simulink model "CSE1_HIL_full16_caseC_new_param"  (R2018b)
settings: Solver=VariableStepAuto  StartTime=0.0  StopTime=300  MaxStep=10e-3  RelTol=1e-3
settings Model: Creator=einarsu  LastModifiedBy=martin
settings OptimizationCC: LifeSpan=inf
settings DebuggingCC: SFExecutionAtInitializationDiag=none
settings SFSimCC: SimUseLocalCustomCode=off
settings RTWCC: RTWUseLocalCustomCode=off
settings CodeAppCC: StateflowObjectComments=on

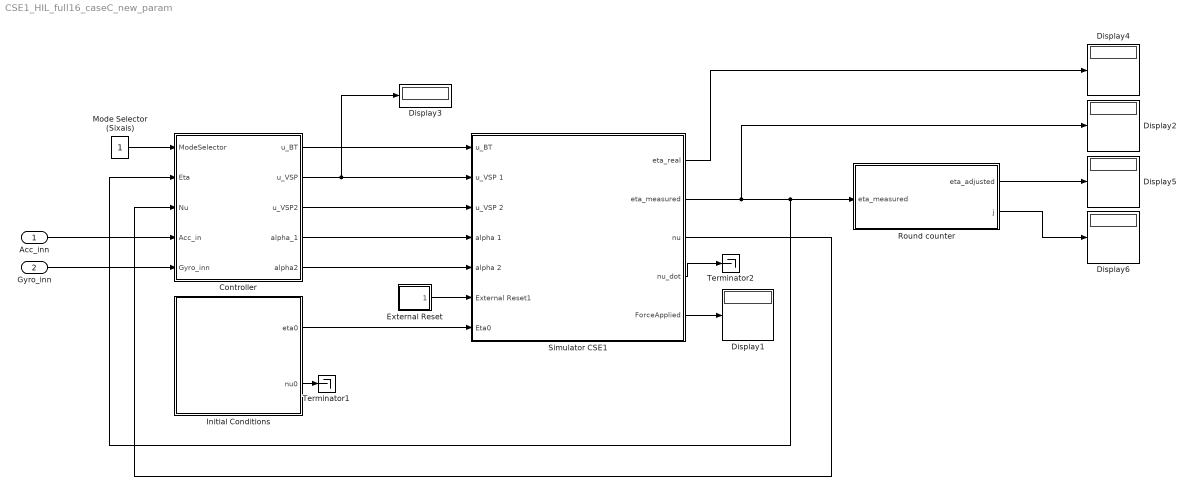
== system CSE1_HIL_full16_caseC_new_param ==
  Acc_inn : Inport
  Gyro_inn : Inport  Port=2
  Controller : Subsystem
  Display{1..6} (6 alike) : Display
  External Reset : Subsystem
  "Initial Conditions " : Subsystem
  Mode Selector (Sixais) : Constant
  Round counter : Subsystem
  Simulator CSE1 : Subsystem
  Terminator1 : Terminator
  Terminator2 : Terminator
  wires:
  Controller/1(u_BT) -> Simulator CSE1/1(u_BT)
  Controller/4(alpha_1) -> Simulator CSE1/4(alpha 1)
  Controller/2(u_VSP) -> Display3/1, Simulator CSE1/2(u_VSP 1)
  Controller/5(alpha2) -> Simulator CSE1/5(alpha 2)
  Controller/3("u_VSP2 ") -> Simulator CSE1/3(u_VSP 2)
  External Reset/1(Out1) -> Simulator CSE1/6(External Reset1)
  "Initial Conditions "/1(eta0) -> Simulator CSE1/7(Eta0)
  Mode Selector (Sixais)/1 -> Controller/1(ModeSelector)
  Simulator CSE1/2(eta_measured) -> Display2/1, Controller/2(Eta), Round counter/1(eta_measured)
  Acc_inn/1 -> Controller/4(Acc_in)
  Gyro_inn/1 -> Controller/5(Gyro_inn)
  Simulator CSE1/5(ForceApplied) -> Display1/1
  "Initial Conditions "/2(nu0) -> Terminator1/1
  Simulator CSE1/4(nu_dot) -> Terminator2/1
  Simulator CSE1/3(nu) -> Controller/3(Nu)
  Simulator CSE1/1(eta_real) -> Display4/1
  Round counter/1(eta_adjusted) -> Display5/1
  Round counter/2(j) -> Display6/1

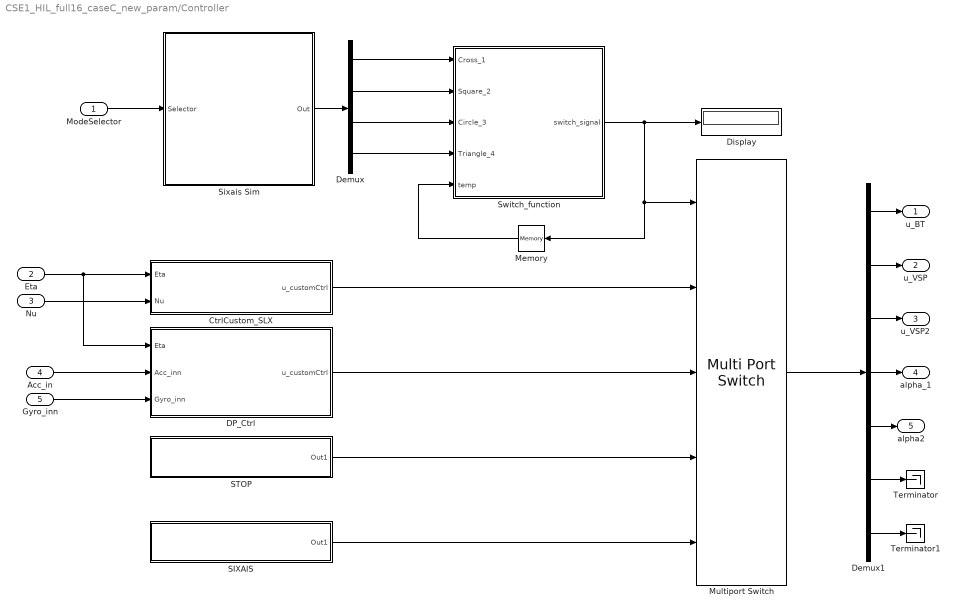
== system CSE1_HIL_full16_caseC_new_param/Controller ==
  ModeSelector : Inport
  Eta : Inport  Port=2
  Nu : Inport  Port=3
  Acc_in : Inport  Port=4
  Gyro_inn : Inport  Port=5
  CtrlCustom_SLX : Subsystem
  DP_Ctrl : Subsystem
  Demux : Demux
  Demux1 : Demux  Outputs=7
  Display : Display
  Memory : Memory  InitialCondition=4
  Multiport Switch : MultiPortSwitch  Inputs=4
  SIXAIS : Subsystem
  STOP : Subsystem
  Sixais Sim : MATLAB Function  TreatAsAtomicUnit=on
  Switch_function : MATLAB Function  TreatAsAtomicUnit=on
  Terminator : Terminator
  Terminator1 : Terminator
  u_BT : Outport
  u_VSP : Outport  Port=2
  "u_VSP2 " : Outport  Port=3
  alpha_1 : Outport  Port=4
  alpha2 : Outport  Port=5
  wires:
  Memory/1 -> Switch_function/5(temp)
  CtrlCustom_SLX/1(u_customCtrl) -> Multiport Switch/2
  Demux/1 -> Switch_function/1(Cross_1)
  Demux/2 -> Switch_function/2(Square_2)
  Demux/3 -> Switch_function/3(Circle_3)
  Demux/4 -> Switch_function/4(Triangle_4)
  Sixais Sim/1(Out) -> Demux/1
  ModeSelector/1 -> Sixais Sim/1(Selector)
  STOP/1(Out1) -> Multiport Switch/4
  SIXAIS/1(Out1) -> Multiport Switch/5
  Eta/1 -> DP_Ctrl/1(Eta), CtrlCustom_SLX/1(Eta)
  Multiport Switch/1 -> Demux1/1
  Demux1/1 -> u_BT/1
  Demux1/2 -> u_VSP/1
  Demux1/3 -> "u_VSP2 "/1
  Demux1/4 -> alpha_1/1
  Demux1/5 -> alpha2/1
  Demux1/6 -> Terminator/1
  Demux1/7 -> Terminator1/1
  Acc_in/1 -> DP_Ctrl/2(Acc_inn)
  Gyro_inn/1 -> DP_Ctrl/3(Gyro_inn)
  DP_Ctrl/1(u_customCtrl) -> Multiport Switch/3
  Switch_function/1(switch_signal) -> Display/1, Memory/1, Multiport Switch/1
  Nu/1 -> CtrlCustom_SLX/2(Nu)

== system CSE1_HIL_full16_caseC_new_param/External Reset ==
  note: Most relevant for Real-Time Simulations...
  Constant : Constant  Value=0
  Out1 : Outport
  wires:
  Constant/1 -> Out1/1

== system CSE1_HIL_full16_caseC_new_param/Initial Conditions  ==
  Eta0 : Constant  Value=[0, 0, 0]'
  "V0 " : Constant  Value=zeros(3,1)
  eta0 : Outport
  nu0 : Outport  Port=2
  wires:
  "V0 "/1 -> nu0/1
  Eta0/1 -> eta0/1

== system CSE1_HIL_full16_caseC_new_param/Round counter ==
  eta_measured : Inport
  Memory : Memory  InitialCondition=[0 0 0]'
  Memory1 : Memory
  Round counter : MATLAB Function  TreatAsAtomicUnit=on
  eta_adjusted : Outport
  j : Outport  Port=2
  wires:
  eta_measured/1 -> Round counter/1(eta_measured)
  Round counter/1(eta_adjusted) -> eta_adjusted/1
  Memory/1 -> Round counter/2(eta_measured_prev)
  Round counter/2(eta_measured_new) -> Memory/1
  Memory1/1 -> Round counter/3(j_prev)
  Round counter/3(j_new) -> Memory1/1, j/1

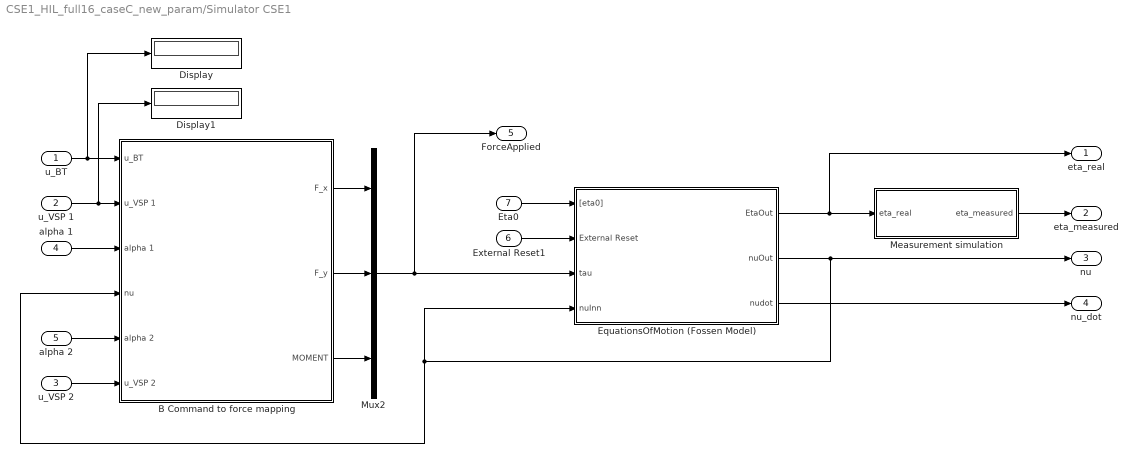
== system CSE1_HIL_full16_caseC_new_param/Simulator CSE1 ==
  u_BT : Inport
  u_VSP 1 : Inport  Port=2
  u_VSP 2 : Inport  Port=3
  alpha 1 : Inport  Port=4
  alpha 2 : Inport  Port=5
  External Reset1 : Inport  Port=6
  Eta0 : Inport  Port=7
  B Command to force mapping : Subsystem
  Display : Display
  Display1 : Display
  EquationsOfMotion (Fossen Model) : Subsystem
  Measurement simulation : MATLAB Function  TreatAsAtomicUnit=on
  Mux2 : Mux  Inputs=3
  eta_real : Outport
  eta_measured : Outport  Port=2
  nu : Outport  Port=3
  nu_dot : Outport  Port=4
  ForceApplied : Outport  Port=5
  wires:
  alpha 2/1 -> B Command to force mapping/5(alpha 2)
  B Command to force mapping/2("F_y ") -> Mux2/2
  B Command to force mapping/1(F_x) -> Mux2/1
  u_VSP 1/1 -> Display1/1, B Command to force mapping/2(u_VSP 1)
  alpha 1/1 -> B Command to force mapping/3(alpha 1)
  u_BT/1 -> Display/1, B Command to force mapping/1(u_BT)
  u_VSP 2/1 -> B Command to force mapping/6(u_VSP 2)
  EquationsOfMotion (Fossen Model)/2(nuOut) -> B Command to force mapping/4(nu), EquationsOfMotion (Fossen Model)/4(nuInn), nu/1
  Eta0/1 -> EquationsOfMotion (Fossen Model)/1("[eta0] ")
  External Reset1/1 -> EquationsOfMotion (Fossen Model)/2(External Reset)
  EquationsOfMotion (Fossen Model)/3(nudot) -> nu_dot/1
  B Command to force mapping/3("MOMENT ") -> Mux2/3
  Mux2/1 -> ForceApplied/1, EquationsOfMotion (Fossen Model)/3(tau)
  EquationsOfMotion (Fossen Model)/1(EtaOut) -> eta_real/1, Measurement simulation/1(eta_real)
  Measurement simulation/1(eta_measured) -> eta_measured/1

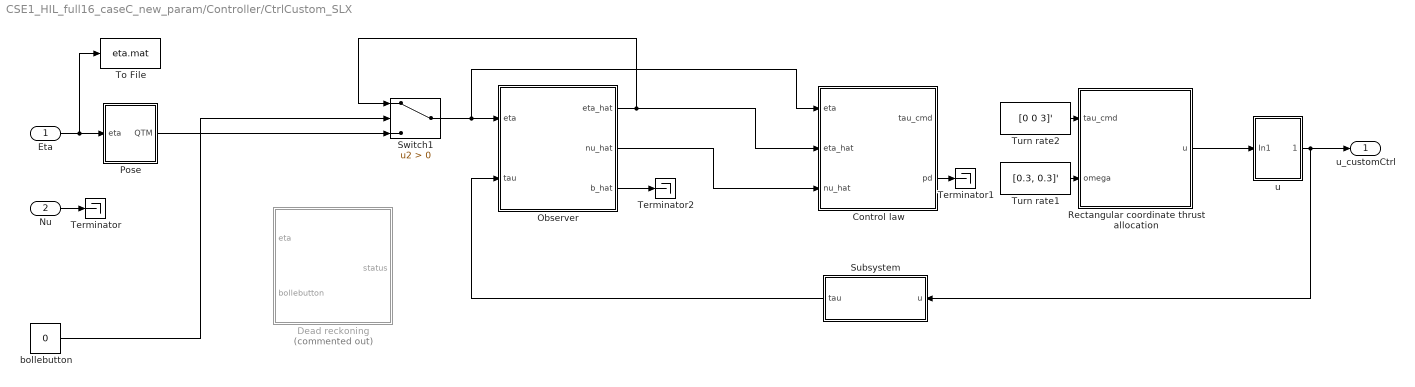
== system CSE1_HIL_full16_caseC_new_param/Controller/CtrlCustom_SLX ==
  Eta : Inport
  Nu : Inport  Port=2
  Control law : Subsystem
  Dead reckoning : Subsystem  Commented=on
  Observer : Subsystem
  Pose : Subsystem
  Rectangular coordinate thrust allocation : Subsystem
  Subsystem : Subsystem
  Switch1 : Switch  Criteria=u2 > Threshold
  Terminator : Terminator
  Terminator1 : Terminator
  Terminator2 : Terminator
  To File : ToFile  Filename=eta.mat  MatrixName=eta
  Turn rate1 : Constant  Value=[0.3, 0.3]'  VectorParams1D=off
  Turn rate2 : Constant  Value=[0 0 3]'  VectorParams1D=off
  bollebutton : Constant  Value=0
  u : Subsystem
  u_customCtrl : Outport
  wires:
  Turn rate1/1 -> Rectangular coordinate thrust allocation/2("omega ")
  Eta/1 -> To File/1, Pose/1(eta)
  u/1(Out1) -> Subsystem/1(u), u_customCtrl/1
  Rectangular coordinate thrust allocation/1(u) -> u/1(In1)
  bollebutton/1 -> Switch1/2
  Pose/1(QTM) -> Switch1/3
  Switch1/1 -> Observer/1(eta), Control law/1(eta)
  Observer/1(eta_hat) -> Control law/2(eta_hat), Switch1/1
  Subsystem/1(tau) -> Observer/2(tau)
  Nu/1 -> Terminator/1
  Observer/2("nu_hat ") -> Control law/3(nu_hat)
  Control law/2(pd) -> Terminator1/1
  Observer/3(b_hat) -> Terminator2/1
  Turn rate2/1 -> Rectangular coordinate thrust allocation/1(tau_cmd)

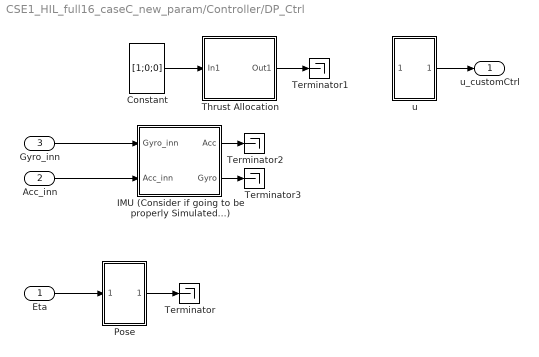
== system CSE1_HIL_full16_caseC_new_param/Controller/DP_Ctrl ==
  Eta : Inport
  Acc_inn : Inport  Port=2
  Gyro_inn : Inport  Port=3
  Constant : Constant  Value=[1;0;0]
  IMU (Consider if going to be properly Simulated...) : Subsystem
  Pose : Subsystem
  Terminator{,1..3} (4 alike) : Terminator
  "Thrust Allocation " : Subsystem
  u : Subsystem
  u_customCtrl : Outport
  wires:
  Pose/1(QTM) -> Terminator/1
  Gyro_inn/1 -> IMU (Consider if going to be properly Simulated...)/1(Gyro_inn)
  Acc_inn/1 -> IMU (Consider if going to be properly Simulated...)/2(Acc_inn)
  Eta/1 -> Pose/1(eta)
  u/1(Out1) -> u_customCtrl/1
  Constant/1 -> "Thrust Allocation "/1(In1)
  "Thrust Allocation "/1(Out1) -> Terminator1/1
  IMU (Consider if going to be properly Simulated...)/1(Acc) -> Terminator2/1
  IMU (Consider if going to be properly Simulated...)/2(Gyro) -> Terminator3/1

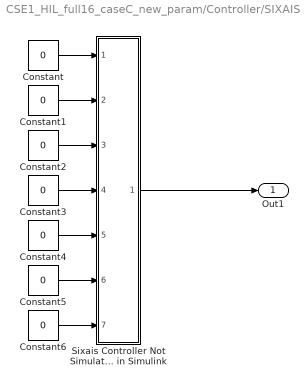
== system CSE1_HIL_full16_caseC_new_param/Controller/SIXAIS ==
  Constant{,1..6} (7 alike) : Constant  Value=0
  Sixais Controller Not Simulated in Simulink : Subsystem
  Out1 : Outport
  wires:
  Constant/1 -> Sixais Controller Not Simulated in Simulink/1(In1)
  Constant1/1 -> Sixais Controller Not Simulated in Simulink/2(In2)
  Constant2/1 -> Sixais Controller Not Simulated in Simulink/3(In3)
  Constant3/1 -> Sixais Controller Not Simulated in Simulink/4(In4)
  Constant4/1 -> Sixais Controller Not Simulated in Simulink/5(In5)
  Constant5/1 -> Sixais Controller Not Simulated in Simulink/6(In6)
  Constant6/1 -> Sixais Controller Not Simulated in Simulink/7(In7)
  Sixais Controller Not Simulated in Simulink/1(Out1) -> Out1/1

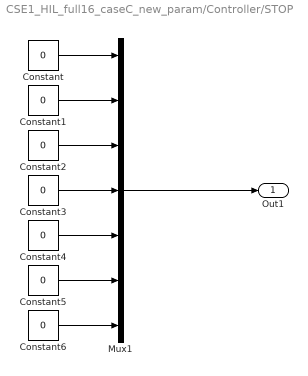
== system CSE1_HIL_full16_caseC_new_param/Controller/STOP ==
  Constant{,1..6} (7 alike) : Constant  Value=0
  Mux1 : Mux  Inputs=7
  Out1 : Outport
  wires:
  Mux1/1 -> Out1/1
  Constant/1 -> Mux1/1
  Constant1/1 -> Mux1/2
  Constant2/1 -> Mux1/3
  Constant3/1 -> Mux1/4
  Constant4/1 -> Mux1/5
  Constant5/1 -> Mux1/6
  Constant6/1 -> Mux1/7

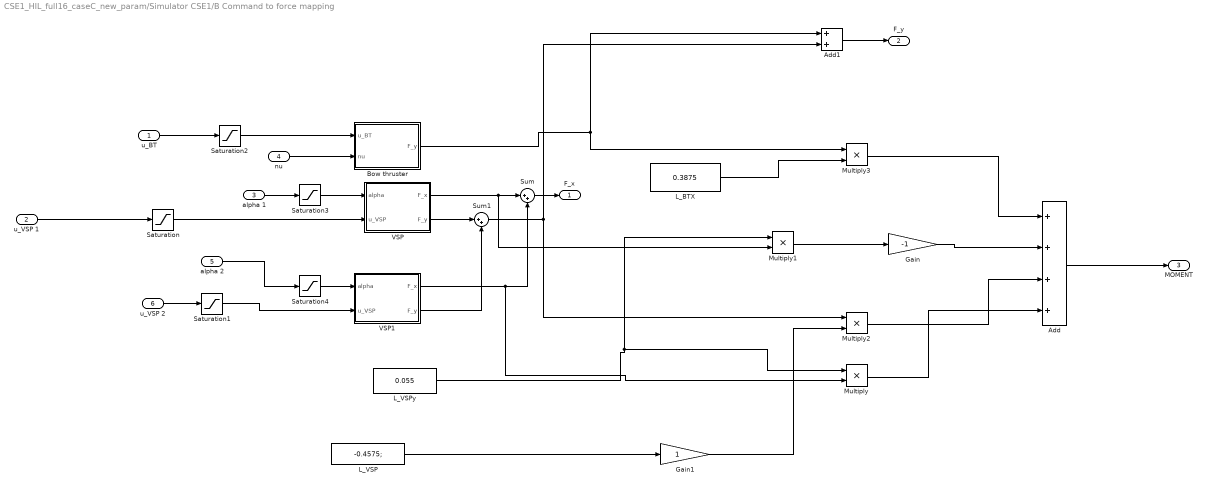
== system CSE1_HIL_full16_caseC_new_param/Simulator CSE1/B Command to force mapping ==
  u_BT : Inport
  u_VSP 1 : Inport  Port=2
  alpha 1 : Inport  Port=3
  nu : Inport  Port=4
  alpha 2 : Inport  Port=5
  u_VSP 2 : Inport  Port=6
  Add : Sum  Inputs=++++
  Add1 : Sum
  Bow thruster : MATLAB Function  TreatAsAtomicUnit=on
  Gain : Gain  Gain=-1
  Gain1 : Gain
  L_BTX : Constant  Value=0.3875
  L_VSP : Constant  Value=-0.4575;
  L_VSPy : Constant  Value=0.055
  Multiply{,1..3} (4 alike) : Product
  Saturation : Saturate  UpperLimit=1  LowerLimit=0
  Saturation1 : Saturate  UpperLimit=1  LowerLimit=0
  Saturation2 : Saturate  UpperLimit=1  LowerLimit=-1
  Saturation3 : Saturate  UpperLimit=pi  LowerLimit=-pi
  Saturation4 : Saturate  UpperLimit=pi  LowerLimit=-pi
  Sum : Sum  Inputs=|++
  Sum1 : Sum  Inputs=|++
  VSP : MATLAB Function  TreatAsAtomicUnit=on
  VSP1 : MATLAB Function  TreatAsAtomicUnit=on
  F_x : Outport
  "F_y " : Outport  Port=2
  "MOMENT " : Outport  Port=3
  wires:
  alpha 1/1 -> Saturation3/1
  nu/1 -> Bow thruster/2(nu)
  Bow thruster/1(F_y) -> Add1/1, Multiply3/1
  VSP/2(F_y) -> Sum1/1
  Sum1/1 -> Add1/2, Multiply2/1
  VSP1/2(F_y) -> Sum1/2
  VSP1/1(F_x) -> Multiply/2, Sum/2
  VSP/1(F_x) -> Multiply1/2, Sum/1
  Sum/1 -> F_x/1
  alpha 2/1 -> Saturation4/1
  u_VSP 2/1 -> Saturation1/1
  L_VSP/1 -> Gain1/1
  L_BTX/1 -> Multiply3/2
  L_VSPy/1 -> Multiply/1, Multiply1/1
  Multiply3/1 -> Add/1
  Multiply1/1 -> Gain/1
  Multiply2/1 -> Add/3
  Multiply/1 -> Add/4
  Add/1 -> "MOMENT "/1
  Gain/1 -> Add/2
  Gain1/1 -> Multiply2/2
  Add1/1 -> "F_y "/1
  Saturation/1 -> VSP/2(u_VSP)
  Saturation1/1 -> VSP1/2(u_VSP)
  u_BT/1 -> Saturation2/1
  u_VSP 1/1 -> Saturation/1
  Saturation2/1 -> Bow thruster/1(u_BT)
  Saturation3/1 -> VSP/1(alpha)
  Saturation4/1 -> VSP1/1(alpha)

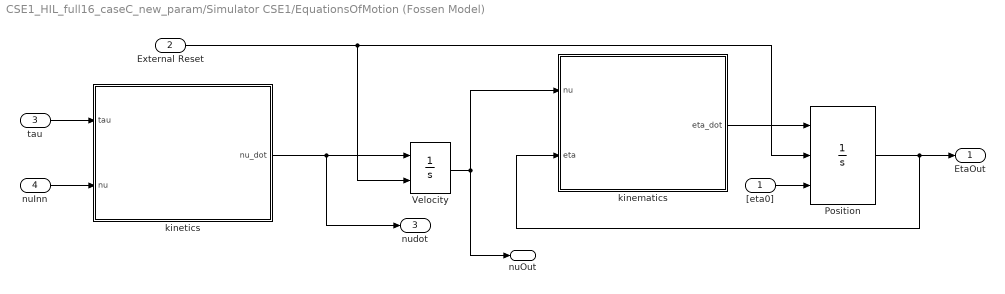
== system CSE1_HIL_full16_caseC_new_param/Simulator CSE1/EquationsOfMotion (Fossen Model) ==
  "[eta0] " : Inport
  External Reset : Inport  Port=2
  tau : Inport  Port=3
  nuInn : Inport  Port=4
  Position : Integrator  ExternalReset=either  InitialConditionSource=external  InitialCondition=[0 0 0]'
  Velocity : Integrator  ExternalReset=either  InitialCondition=[0 0 0]'
  kinematics : MATLAB Function  TreatAsAtomicUnit=on
  kinetics : MATLAB Function  TreatAsAtomicUnit=on
  EtaOut : Outport
  nuOut : Outport  Port=2
  nudot : Outport  Port=3
  wires:
  tau/1 -> kinetics/1(tau)
  Position/1 -> kinematics/2(eta), EtaOut/1
  "[eta0] "/1 -> Position/3
  nuInn/1 -> kinetics/2(nu)
  kinematics/1(eta_dot) -> Position/1
  Velocity/1 -> kinematics/1(nu), nuOut/1
  kinetics/1(nu_dot) -> nudot/1, Velocity/1
  External Reset/1 -> Position/2, Velocity/2

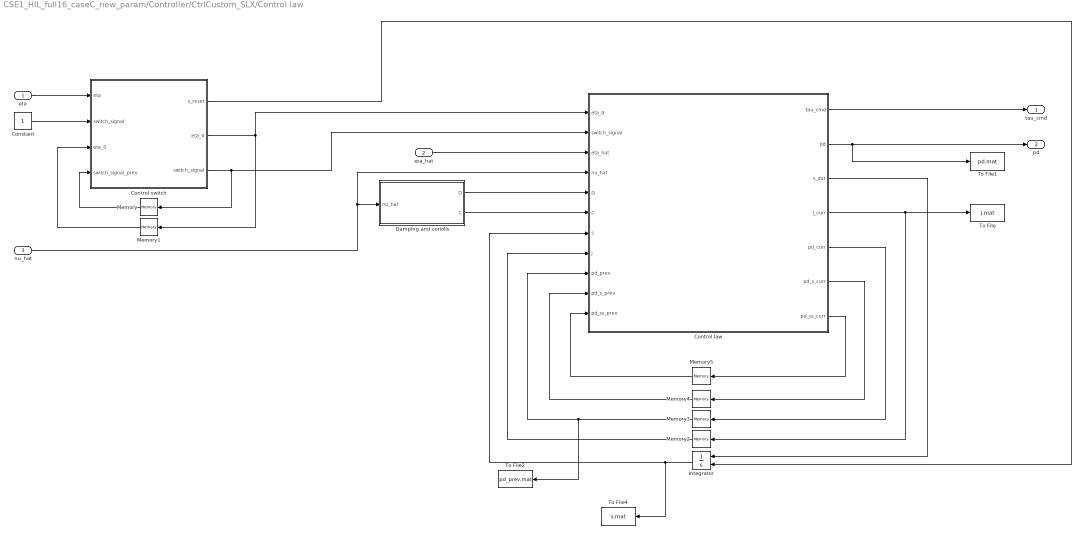
== system CSE1_HIL_full16_caseC_new_param/Controller/CtrlCustom_SLX/Control law ==
  eta : Inport
  eta_hat : Inport  Port=2
  nu_hat : Inport  Port=3
  " Control switch" : MATLAB Function  TreatAsAtomicUnit=on
  Constant : Constant
  Control law : MATLAB Function  TreatAsAtomicUnit=on
  Damping and coriolis : MATLAB Function  TreatAsAtomicUnit=on
  Integrator : Integrator  ExternalReset=either
  Memory : Memory
  Memory1 : Memory  InitialCondition=[0, 0, 0]'
  Memory2 : Memory
  Memory3 : Memory  InitialCondition=[0;0;0]
  Memory4 : Memory  InitialCondition=[0;0;0]
  Memory5 : Memory  InitialCondition=[0;0;0]
  To File : ToFile  Filename=j.mat  MatrixName=j
  To File1 : ToFile  Filename=pd.mat  MatrixName=pd
  To File2 : ToFile  Filename=pd_prev.mat  MatrixName=pd_prev
  To File4 : ToFile  Filename=s.mat  MatrixName=s
  tau_cmd : Outport
  pd : Outport  Port=2
  wires:
  " Control switch"/2(eta_0) -> Memory1/1, Control law/1(eta_0)
  Integrator/1 -> To File4/1, Control law/7(s)
  Damping and coriolis/1(D) -> Control law/5(D)
  Control law/3(s_dot) -> Integrator/1
  Memory1/1 -> " Control switch"/3("eta_0 ")
  " Control switch"/3(switch_signal) -> Memory/1, Control law/2(switch_signal)
  Memory/1 -> " Control switch"/4(switch_signal_prev)
  eta/1 -> " Control switch"/1(eta)
  Constant/1 -> " Control switch"/2("switch_signal ")
  Control law/2(pd) -> To File1/1, pd/1
  Control law/1(tau_cmd) -> tau_cmd/1
  nu_hat/1 -> Damping and coriolis/1(nu_hat), Control law/4(nu_hat)
  Control law/4(j_curr) -> Memory2/1, To File/1
  Memory2/1 -> Control law/8(j)
  Memory3/1 -> Control law/9(pd_prev), To File2/1
  Control law/5(pd_curr) -> Memory3/1
  Damping and coriolis/2(C) -> Control law/6(C)
  eta_hat/1 -> Control law/3(eta_hat)
  Control law/6(pd_s_curr) -> Memory4/1
  Control law/7(pd_ss_curr) -> Memory5/1
  Memory5/1 -> Control law/11(pd_ss_prev)
  Memory4/1 -> Control law/10(pd_s_prev)
  " Control switch"/1(s_reset) -> Integrator/2

== system CSE1_HIL_full16_caseC_new_param/Controller/CtrlCustom_SLX/Dead reckoning ==
  eta : Inport
  bollebutton : Inport  Port=2
  Display : Display
  Memory : Memory  InitialCondition=[0 0 0]'
  Memory1 : Memory  InitialCondition=[0 0 0]'
  Memory2 : Memory  InitialCondition=[0 0 0]'
  dead_reckoning : MATLAB Function  TreatAsAtomicUnit=on
  status : Outport
  wires:
  Memory2/1 -> dead_reckoning/3("last ")
  Memory/1 -> dead_reckoning/5("last3 ")
  dead_reckoning/3(last2) -> Memory1/1
  dead_reckoning/4(last3) -> Memory/1
  Memory1/1 -> dead_reckoning/4("last2 ")
  dead_reckoning/2(last) -> Memory2/1
  eta/1 -> dead_reckoning/1(eta)
  bollebutton/1 -> dead_reckoning/2(bollebutton)
  dead_reckoning/1(status) -> Display/1, status/1

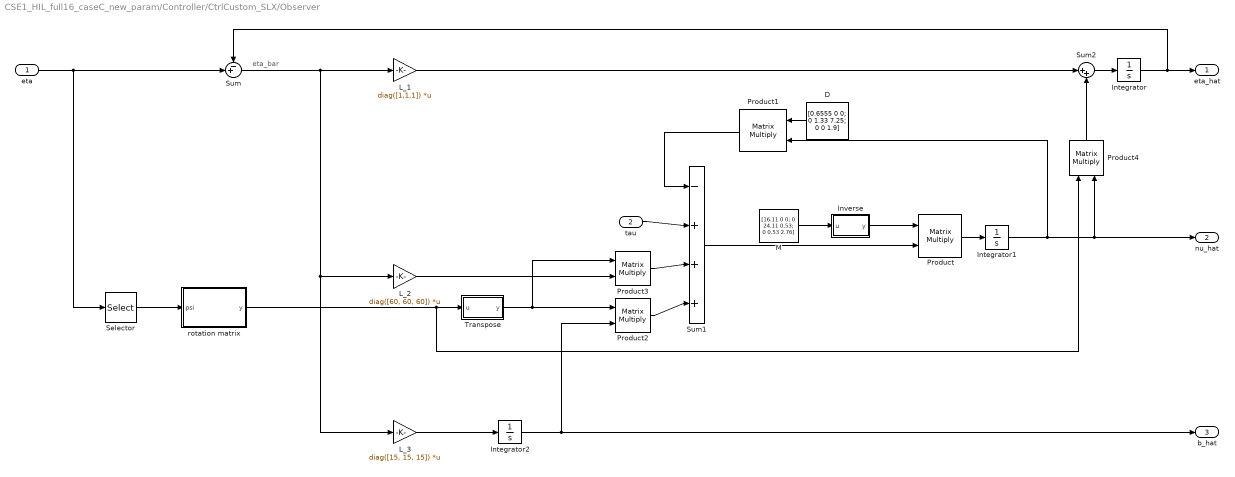
== system CSE1_HIL_full16_caseC_new_param/Controller/CtrlCustom_SLX/Observer ==
  note: eta_bar
  eta : Inport
  tau : Inport  Port=2
  D : Constant  Value=[0.6555 0 0; 0 1.33 7.25; 0 0 1.9]
  Integrator : Integrator  InitialCondition=[0 0 0]'
  Integrator1 : Integrator  InitialCondition=[0 0 0]'  UpperSaturationLimit=1000  LowerSaturationLimit=-1000
  Integrator2 : Integrator
  Inverse : MATLAB Function  TreatAsAtomicUnit=on
  L_1 : Gain  Gain=diag([1,1,1])  Multiplication=Matrix(K*u)
  L_2 : Gain  Gain=diag([60, 60, 60])  Multiplication=Matrix(K*u)
  L_3 : Gain  Gain=diag([15, 15, 15])  Multiplication=Matrix(K*u)
  M : Constant  Value=[16.11 0 0; 0 24.11 0.53; 0 0.53 2.76]
  Product{,1..4} (5 alike) : Product  Multiplication=Matrix(*)
  Selector : Selector  InputPortWidth=3  IndexOptions=Index vector (dialog)  Indices=[3]  OutputSizes=1
  Sum : Sum  Inputs=-+|
  Sum1 : Sum  Inputs=-|+|+|+
  Sum2 : Sum  Inputs=|++
  Transpose : MATLAB Function  TreatAsAtomicUnit=on
  rotation matrix : MATLAB Function  TreatAsAtomicUnit=on
  eta_hat : Outport
  "nu_hat " : Outport  Port=2
  b_hat : Outport  Port=3
  wires:
  Sum/1 -> L_3/1, L_2/1, L_1/1
  eta/1 -> Selector/1, Sum/2
  Selector/1 -> rotation matrix/1(psi)
  Integrator/1 -> eta_hat/1, Sum/1
  Inverse/1(y) -> Product/1
  M/1 -> Inverse/1(u)
  D/1 -> Product1/1
  Product1/1 -> Sum1/1
  rotation matrix/1(y) -> Product4/1, Transpose/1(u)
  Transpose/1(y) -> Product3/1, Product2/1
  L_2/1 -> Product3/2
  Sum1/1 -> Product/2
  Product/1 -> Integrator1/1
  L_1/1 -> Sum2/1
  Product4/1 -> Sum2/2
  Sum2/1 -> Integrator/1
  Integrator1/1 -> Product1/2, Product4/2, "nu_hat "/1
  L_3/1 -> Integrator2/1
  Integrator2/1 -> b_hat/1, Product2/2
  Product3/1 -> Sum1/3
  tau/1 -> Sum1/2
  Product2/1 -> Sum1/4

== system CSE1_HIL_full16_caseC_new_param/Controller/CtrlCustom_SLX/Pose ==
  eta : Inport
  Demux : Demux  Outputs=3
  Mux : Mux  Inputs=3
  QTM : Outport
  wires:
  eta/1 -> Demux/1
  Mux/1 -> QTM/1
  Demux/1 -> Mux/1  "x_m"
  Demux/3 -> Mux/3  "psi_m"
  Demux/2 -> Mux/2  "y_m"

== system CSE1_HIL_full16_caseC_new_param/Controller/CtrlCustom_SLX/Rectangular coordinate thrust allocation ==
  tau_cmd : Inport
  "omega " : Inport  Port=2
  Demux : Demux  Outputs=5
  Demux1 : Demux  Outputs=2
  MATLAB Function : MATLAB Function  TreatAsAtomicUnit=on
  Mux : Mux  Inputs=7
  Selector : Selector  InputPortWidth=5  IndexOptions=Index vector (dialog)  Indices=[3 1 2 4 5]  OutputSizes=1
  u : Outport
  wires:
  Mux/1 -> u/1
  Demux1/1 -> Mux/6
  Demux1/2 -> Mux/7
  Demux/5 -> Mux/5
  Demux/4 -> Mux/4
  "omega "/1 -> Demux1/1
  MATLAB Function/1(u_ext) -> Selector/1
  tau_cmd/1 -> MATLAB Function/1(tau_cmd)
  Demux/1 -> Mux/1
  Demux/2 -> Mux/2
  Demux/3 -> Mux/3
  Selector/1 -> Demux/1

== system CSE1_HIL_full16_caseC_new_param/Controller/CtrlCustom_SLX/Subsystem ==
  u : Inport
  u_to_tau_mapping : MATLAB Function  TreatAsAtomicUnit=on
  tau : Outport
  wires:
  u/1 -> u_to_tau_mapping/1(u_ext)
  u_to_tau_mapping/1(tau) -> tau/1

== system CSE1_HIL_full16_caseC_new_param/Controller/CtrlCustom_SLX/u ==
  In1 : Inport
  Demux1 : Demux  Outputs=7
  Mux : Mux  Inputs=7
  Saturation1 : Saturate  UpperLimit=1  LowerLimit=0
  Saturation11 : Saturate  UpperLimit=1  LowerLimit=0
  Saturation2 : Saturate  UpperLimit=1  LowerLimit=-1
  Out1 : Outport
  wires:
  Saturation1/1 -> Mux/3
  Saturation11/1 -> Mux/2
  Mux/1 -> Out1/1
  Demux1/7 -> Mux/7  "omega_VSP2"
  Demux1/6 -> Mux/6  "omega_VSP1"
  Demux1/5 -> Mux/5  "alpha_VSP2"
  Demux1/4 -> Mux/4  "alpha_VSP1"
  Demux1/3 -> Saturation1/1  "u_VSP2"
  Demux1/2 -> Saturation11/1  "u_VSP1"
  Demux1/1 -> Saturation2/1  "u_BT"
  In1/1 -> Demux1/1
  Saturation2/1 -> Mux/1

== system CSE1_HIL_full16_caseC_new_param/Controller/DP_Ctrl/IMU (Consider if going to be properly Simulated...) ==
  Gyro_inn : Inport
  Acc_inn : Inport  Port=2
  Demux : Demux  Outputs=3
  Demux1 : Demux  Outputs=3
  Mux : Mux  Inputs=3
  Mux2 : Mux  Inputs=3
  Acc : Outport
  Gyro : Outport  Port=2
  wires:
  Acc_inn/1 -> Demux1/1
  Gyro_inn/1 -> Demux/1
  Demux/1 -> Mux2/1
  Demux/2 -> Mux2/2
  Demux/3 -> Mux2/3
  Demux1/2 -> Mux/2
  Demux1/3 -> Mux/3
  Mux2/1 -> Gyro/1
  Demux1/1 -> Mux/1
  Mux/1 -> Acc/1

== system CSE1_HIL_full16_caseC_new_param/Controller/DP_Ctrl/Pose ==
  eta : Inport
  Demux : Demux  Outputs=3
  Mux : Mux  Inputs=3
  QTM : Outport
  wires:
  eta/1 -> Demux/1
  Mux/1 -> QTM/1
  Demux/1 -> Mux/1  "x_m"
  Demux/3 -> Mux/3  "psi_m"
  Demux/2 -> Mux/2  "y_m"

== system CSE1_HIL_full16_caseC_new_param/Controller/DP_Ctrl/Thrust Allocation  ==
  In1 : Inport
  THALOC (u->tau) : MATLAB Function  TreatAsAtomicUnit=on
  Out1 : Outport
  wires:
  In1/1 -> THALOC (u->tau)/1(u)
  THALOC (u->tau)/1(y) -> Out1/1

== system CSE1_HIL_full16_caseC_new_param/Controller/DP_Ctrl/u ==
  In1 : Inport
  Demux1 : Demux  Outputs=7
  Mux : Mux  Inputs=7
  Out1 : Outport
  wires:
  Mux/1 -> Out1/1
  Demux1/7 -> Mux/7  "omega_VSP2"
  Demux1/6 -> Mux/6  "omega_VSP1"
  Demux1/5 -> Mux/5  "alpha_VSP2"
  Demux1/4 -> Mux/4  "alpha_VSP1"
  Demux1/3 -> Mux/3  "u_VSP2"
  Demux1/2 -> Mux/2  "u_VSP1"
  Demux1/1 -> Mux/1  "u_BT"
  In1/1 -> Demux1/1

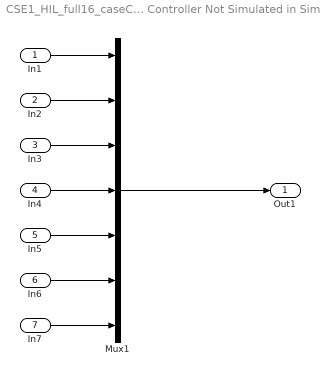
== system CSE1_HIL_full16_caseC_new_param/Controller/SIXAIS/Sixais Controller Not Simulated in Simulink ==
  In1 : Inport
  In2 : Inport  Port=2
  In3 : Inport  Port=3
  In4 : Inport  Port=4
  In5 : Inport  Port=5
  In6 : Inport  Port=6
  In7 : Inport  Port=7
  Mux1 : Mux  Inputs=7
  Out1 : Outport
  wires:
  In4/1 -> Mux1/4
  In5/1 -> Mux1/5
  In6/1 -> Mux1/6
  In3/1 -> Mux1/3
  In1/1 -> Mux1/1
  In2/1 -> Mux1/2
  Mux1/1 -> Out1/1
  In7/1 -> Mux1/7

== matlab function CSE1_HIL_full16_caseC_new_param/Simulator CSE1/EquationsOfMotion (Fossen Model)/kinematics ==
  data: nu input; eta_dot output; eta input
function eta_dot = CSE1_eta_dot(nu,eta)

psi = eta(3);

J = [cos(psi) -sin(psi) 0
     sin(psi) cos(psi)  0
     0        0         1];

eta_dot = J*nu;

== matlab function CSE1_HIL_full16_caseC_new_param/Simulator CSE1/EquationsOfMotion (Fossen Model)/kinetics ==
  data: tau input; nu_dot output; nu input
function nu_dot = CSE1_nu_dot(tau,nu)

u   = nu(1);
v   = nu(2);
r   = nu(3);

tau = [tau(1);tau(2);tau(3)];
%% MATRICES 
%changed m from 14.79 to 14.11

m    = 14.11;   I_z  =  1.7600;   x_g = 0.0375;       % x_g  =  0.0460; % Table B.1

%% Added mass
%changed Y_vd from -1.0 to -10.0
X_ud  =     -2.0;											% Table B.1
					Y_vd =      -10.0;	N_vd =    -0.0;		% Table B.1
					Y_rd =      -0.0;	N_rd =    -1.0;		% Table B.1

%% Total mass matrix
m_11 = m-X_ud;
m_22 = m-Y_vd;
m_23 = m*x_g-Y_rd;
m_32 = m*x_g-N_vd; % noted as Y_rd in handbook, but same value
m_33 = I_z-N_rd;

M    = [m_11 0    0
        0    m_22 m_23
        0    m_32 m_33];
	
%% Damping coefficients
% Comments at the end of the lines indicate the old values used.
X_u		= -0.6555;		X_v		= 0;
X_uu 	= 0.3545;		X_vv	= -2.443;
X_uuu 	= -3.787;		X_vvv	= 0;

						Y_v		= -1.33; 			Y_r		= -7.250; % Y_r
						Y_vv	= -2.776;			Y_rr	= -3.450; % Y_rr
						Y_vvv	= -64.91;			Y_rrr	= 0;
						
						Y_rv	= -0.805;			Y_vr	= -0.845; % Y_rv, Y_vr

						N_v		= 0;				N_r		= -1.900; % N_r
						N_vv	= -0.2088;			N_rr	= -0.750; % N_rr
						N_vvv	= 0;				N_rrr	= 0;
						
						N_rv	= 0.130;			N_vr	= 0.080; % N_rv, N_vr

%% Correolis matrix
c_13 = -(m-Y_vd)*v-(m*x_g-Y_rd)*r;
c_23 = (m-X_ud)*u;
C    = [0     0     c_13
        0     0     c_23
        -c_13 -c_23 0   ];

%% Assembly of the damping matrix
%should be abs(u), abs(v) some places, only positive values? 

d_11 = -X_u - X_uu*u - X_uuu*u^2;
d_22 = -Y_v - Y_vv*v - Y_vvv*v^2 - Y_rv*abs(r);
d_33 = -N_r - N_rr*abs(r) - N_rrr*r^2 - N_vr*abs(v); % using abs(r)

d_12 = -X_v - X_vv*v - X_vvv*v^2;
d_23 = -Y_r - Y_rr*abs(r) - Y_rrr*r^2 - Y_vr*abs(v);
d_32 = -N_v - N_vv*v - N_vvv*v^2 - N_rv*abs(r);

%D    = [d_11 d_12 0      vet ikke hvorfor d_12 er her
%        0    d_22 d_23
%        0    d_32 d_33];
D    = [d_11 0 0
        0    d_22 d_23
        0    d_32 d_33];


%% CALCULATION
nu_dot = M\(tau-(C+D)*nu);

== matlab function CSE1_HIL_full16_caseC_new_param/Controller/CtrlCustom_SLX/Control law/ Control switch ==
  data: s_reset output; eta_0 output; eta input; switch_signal output; switch_signal input; eta_0 input; switch_signal_prev input
function [s_reset,eta_0,switch_signal] = control_switch(eta,switch_signal,eta_0,switch_signal_prev)

if switch_signal ~= 0 && switch_signal_prev == 0
    eta_0 = eta;
    s_reset = 1;
else
    s_reset = 0;
end

%s_reset = 0;

== matlab function CSE1_HIL_full16_caseC_new_param/Controller/CtrlCustom_SLX/Dead reckoning/dead_reckoning ==
  data: eta input; bollebutton input; status output; last input; last output; last2 output; last3 output; last2 input; last3 input
function [status, last, last2, last3] = dead_reckoning(eta, bollebutton, last, last2, last3)

if (eta(1) == last(1) && eta(2) == last(2) && eta(3) == last(3) && ...
        eta(1) == last2(1) && eta(2) == last2(2) && eta(3) == last2(3) ...
       && eta(1) == last3(1) && eta(2) == last3(2) && eta(3) == last3(3))
    status = 0;
else
    status = 1;
end

if bollebutton == 1
    status = 0;
end
   
last3 = last2;
last2 = last;
last = eta;
end

== matlab function CSE1_HIL_full16_caseC_new_param/Controller/CtrlCustom_SLX/Rectangular coordinate thrust allocation/MATLAB Function ==
  data: tau_cmd input; u_ext output
function u_ext = fcn(tau_cmd)

%%
%Initialize extended thrust allocation matrix
L_xvsp = 0.4574;
L_yvsp = 0.055;
L_bt = 0.3875;

L_xvsp_1 = -L_xvsp;
L_yvsp_1 = -L_yvsp;
L_xvsp_2 = -L_xvsp;
L_yvsp_2 = L_yvsp;

B_ext = [1         0        1         0        0;
         0         1        0         1        1;
        -L_yvsp_1  L_xvsp_1 -L_yvsp_2 L_xvsp_2 L_bt];
 
B_ext_inv = pinv(B_ext);

%Extended force vector
f = B_ext_inv*tau_cmd;

%%
%Calculate angles and control input
alpha_1 = atan2(f(2), f(1));
alpha_2 = atan2(f(4), f(3));

alpha = [alpha_1; alpha_2];

k_1 = 1.03;
k_2 = 1.03;
k_3 = 2.629;

u_1 = (1/k_2)*sqrt(f(1)^2 + f(2)^2);
u_2 = (1/k_3)*sqrt(f(3)^2 + f(4)^2);
u_3 = f(5)/k_1;

u = [u_1; u_2; u_3];

u_ext = [u; alpha];

== matlab function CSE1_HIL_full16_caseC_new_param/Controller/CtrlCustom_SLX/Control law/Control law ==
  data: eta_0 input; switch_signal input; eta_hat input; nu_hat input; D input; C input; s input; j input; pd_prev input; pd_s_prev input; tau_cmd output; pd output; s_dot output; j_curr output; pd_curr output; pd_ss_prev input; pd_s_curr output; pd_ss_curr output
function [tau_cmd, pd, s_dot, j_curr, pd_curr, pd_s_curr, pd_ss_curr] ...
    = control_law( ...
    eta_0, switch_signal, eta_hat, nu_hat, D, C, s, ...
    j, pd_prev, pd_s_prev, pd_ss_prev)
%% Path parameters

path = "ellipsoidal"; % "linear" or "ellipsoidal"
div_zero_const = 1e-3;

rx  = 4;
ry  = 4;

%% Control law parameters

mu = 0.001;
U_ref = 0.1;

Kp = diag([0.2 0.2 0.1]);
Kd = diag([10 10 5]);

%% Starting point conditions

p_0   = [   eta_0(1);
            eta_0(2)];
        
p_1   = [   p_0(1) + cos(eta_0(3));
            p_0(2) + sin(eta_0(3))];

p_c   = [   p_0(1);
            p_0(2) + ry];

%% Rotation and rotation speed matrices

Rot_mat = [cos(eta_hat(3))  -sin(eta_hat(3))    0;
           sin(eta_hat(3))  cos(eta_hat(3))     0;
           0                0                   1];

S_mat = [0          -nu_hat(3)  0;
         nu_hat(3)  0           0;
         0          0           0];

%% Path parameterization

if path == "linear"
    p_x = p_0(1) + (p_1(1) - p_0(1))*s;
    p_y = p_0(2) + (p_1(2) - p_0(2))*s;
    p_x_s = p_1(1) - p_0(1);
    p_y_s = p_1(2) - p_0(2);
    p_x_ss = 0;
    p_y_ss = 0;
    p_x_sss = 0;
    p_y_sss = 0;
elseif path == "ellipsoidal"
    p_x = p_c(1) + rx*sin(2*pi*s);
    p_y = p_c(2) - ry*cos(2*pi*s);
    p_x_s = 2*pi*rx*cos(2*pi*s);
    p_y_s = 2*pi*ry*sin(2*pi*s);
    p_x_ss = -(2*pi)^2*rx*sin(2*pi*s);
    p_y_ss = (2*pi)^2*ry*cos(2*pi*s);
    p_x_sss = -(2*pi)^3*rx*cos(2*pi*s);
    p_y_sss = -(2*pi)^3*ry*sin(2*pi*s);
elseif path == "4-corner"
    p_x = 0;
    p_y = 0;
    p_x_s = 0;
    p_y_s = 0;
    p_x_ss = 0;
    p_y_ss = 0;
    p_x_sss = 0;
    p_y_sss = 0;
else
    p_x = 0;
    p_y = 0;
    p_x_s = 0;
    p_y_s = 0;
    p_x_ss = 0;
    p_y_ss = 0;
    p_x_sss = 0;
    p_y_sss = 0;
end

%% Division by zero prevention

if p_x_s == 0 && p_y_s == 0
    if pd_s_prev(1) ~= 0
        p_x_s = pd_s_prev(1);
    else
        p_x_s = div_zero_const;
    end
    if pd_s_prev(2) ~= 0
        p_y_s = pd_s_prev(2);
    else
        p_y_s = div_zero_const;
    end
end

if (p_x_ss + p_y_ss) == 0
    if (pd_ss_prev(1) + pd_ss_prev(2)) ~= 0
        p_x_ss = pd_ss_prev(1);
        p_y_ss = pd_ss_prev(2);
    else
        p_x_ss = div_zero_const / 2;
        p_y_ss = div_zero_const / 2;
    end
end

%% Calculate path vectors

pd      = [ p_x;
            p_y;
            atan2(p_y_s, p_x_s)];
pd_s    = [ p_x_s;
            p_y_s;
            (p_x_s*p_y_ss - p_y_s*p_x_ss) / (p_x_ss + p_y_ss)];
pd_ss   = [ p_x_ss;
            p_y_ss;
            (p_x_s*p_y_sss - p_y_s*p_x_sss) / ((p_x_s)^2 + (p_y_s)^2) ...
            - 2 * (p_x_s*p_y_ss - p_y_s*p_x_ss) ...
            * (p_x_s*p_x_ss + p_y_s*p_y_ss) / ((p_x_s)^2 + (p_y_s)^2)^2];

%% Making atan2 continuous

% If jump from positive Q2 to neg Q3
if (pd(3,1) - (pd_prev(3,1)-2*pi*j)) < -pi ...
        && (pd(3,1)-(pd_prev(3,1)-2*pi*j)) >= -2*pi
    j = j + 1;
% If jump from negative Q3 to pos Q2
elseif (pd(3,1) - (pd_prev(3,1)-2*pi*j)) > pi ...
        && (pd(3,1)-(pd_prev(3,1)-2*pi*j)) <= 2*pi
    j = j - 1;
end

pd(3,1) = 2*pi*j + pd(3,1);

%% Update laws

Us    = U_ref / norm(pd_s);

z1 = Rot_mat'*(eta_hat - pd);
V_s   = -(eta_hat-pd)'*pd_s;
omega = mu*V_s / norm(pd_s);

s_dot = (Us - omega);

Us_s  = (-U_ref*((pd_s(1)*pd_ss(1))+(pd_s(2)*pd_ss(2)))) ...
        / (pd_s(1)^2 + pd_s(2)^2)^(3/2);
Us_dot = Us_s * s_dot;


alpha1 = -Kp*z1 + pd_s*Us;

%% Control law

% Include bias and coriolis matrix?
M = [16.11 0 0; 0 24.11 0.53; 0 0.53 2.76];

alpha1_dot = ...
    Kp*(S_mat*z1 - nu_hat) ...
    - S_mat*Rot_mat'*pd_s*Us ...
    + Rot_mat'*pd_s*Us_dot ...
    + (Kp*Rot_mat'*pd_s + Rot_mat'*(pd_ss*Us + pd_s*Us_s))*s_dot;

z2 = nu_hat - alpha1;

%% Switch logics

if switch_signal~=0
    tau_cmd = -z1 + D*nu_hat + C*nu_hat + M*alpha1_dot - Kd*z2;
else
    tau_cmd = zeros(3,1);
end

%% Assign variables for memory blocks

j_curr = j;
pd_curr = pd;
pd_s_curr = pd_s;
pd_ss_curr = pd_ss;

end

== matlab function CSE1_HIL_full16_caseC_new_param/Controller/CtrlCustom_SLX/Observer/rotation matrix ==
  data: psi input; y output
function y = rotation_matrix(psi)

y = [cos(psi) -sin(psi) 0;
    sin(psi) cos(psi) 0;
    0 0 1];
 end

== matlab function CSE1_HIL_full16_caseC_new_param/Controller/Switch_function ==
  data: Cross_1 input; switch_signal output; Square_2 input; Circle_3 input; Triangle_4 input; temp input
%% Function that takes in impulse button sigals [0,1] and sends out a 
% different signal depentent pn which button has been pressed

function switch_signal = fcn(Cross_1,Square_2,Circle_3,Triangle_4,temp)
%#codegen
persistent signal;

signal = temp;

if Cross_1 ~= 0
    signal = 1;
end

if Square_2 ~= 0
    signal = 2;
end

if Circle_3 ~= 0
    signal = 3;
end
    
if Triangle_4 ~= 0
    signal = 4; 
end

switch_signal = signal;

== matlab function CSE1_HIL_full16_caseC_new_param/Controller/Sixais Sim ==
  data: Selector input; Out output
%% Function that takes in impulse button sigals [0,1] and sends out a 
% different signal depentent pn which button has been pressed

function Out = fcn(Selector)
%#codegen
if Selector==1
    Out=[1 0 0 0];
elseif Selector==2
        Out=[0 1 0 0];
elseif Selector==4
        Out=[0 0 0 1];
else 
        Out=[0 0 1 0];

end

== matlab function CSE1_HIL_full16_caseC_new_param/Controller/DP_Ctrl/Thrust Allocation /THALOC (u->tau) ==
  data: u input; y output
function y = fcn(u)

y = u;

== matlab function CSE1_HIL_full16_caseC_new_param/Controller/CtrlCustom_SLX/Subsystem/u_to_tau_mapping ==
  data: u_ext input; tau output
function tau = fcn(u_ext)

%% Thruster configuration
Lx_vsp = 0.4574;
Ly_vsp = 0.055;
Lx_bt = 0.3875;

Lx_vsp_1 = -Lx_vsp;
Ly_vsp_1 = -Ly_vsp;
Lx_vsp_2 = -Lx_vsp;
Ly_vsp_2 = Ly_vsp;

k_1 = 1.03;
k_2 = 1.03;
k_3 = 2.629;

K = diag([k_3 k_1 k_2]);

u = u_ext(1:3);

%% Mapping
alpha_vsp1 = u_ext(4);
alpha_vsp2 = u_ext(5);

B = [0          cos(alpha_vsp1)         cos(alpha_vsp2);
     1          sin(alpha_vsp1)         sin(alpha_vsp2);
     Lx_bt       Lx_vsp_1*sin(alpha_vsp1)-Ly_vsp_1*cos(alpha_vsp1)   Lx_vsp_2*sin(alpha_vsp2)-Ly_vsp_2*cos(alpha_vsp2)];
    
tau = B*K*u;
end

== matlab function CSE1_HIL_full16_caseC_new_param/Simulator CSE1/B Command to force mapping/Bow thruster ==
  data: u_BT input; F_y output; nu input
function F_y = fcn(u_BT,nu)
%#codegen
u = nu(1);
% Thruster characteristics
if u_BT >0
    u_BT=u_BT+ 0.059;
    a =        -548;
    b =       0.193;
    c =       548.2;
    d =      0.1992;
    y0 = -(a*exp(b*-u_BT) + c*exp(d*-u_BT));
elseif u_BT < 0
    u_BT=u_BT- 0.059;
    a =        -548;
    b =       0.193;
    c =       548.2;
    d =      0.1992;
    y0 = a*exp(b*u_BT) + c*exp(d*u_BT);
else
    y0 = 0;
end
% Thruster losses due to forward speed
a0 =      0.7561;
a1 =      0.3075;
b1 =      -10.22;
c1 =       2.947;
F_y = y0*(a0 + a1*atan(b1*u +c1))/1.1385;
F_y=F_y*2.62/2.7629;


%2019 changes- Some add-hock changes, because it did not make sense previously.

== matlab function CSE1_HIL_full16_caseC_new_param/Simulator CSE1/B Command to force mapping/VSP ==
  data: alpha input; F_x output; u_VSP input; F_y output
function [ F_x , F_y ] = fcn(alpha,u_VSP)
%#codegen
% Calculating the force in x-direction
a1 =       1.107  ;
b1 =       1.001  ;
c1 =       1.564  ;
a2 =      0.3471 ;
b2 =      0.1397 ;
c2 =      -1.599  ;
a3 =      0.1558 ;
b3 =       1.993  ;
c3 =       1.886  ;
a4 =      0.1599 ;
b4 =       0.218  ;
c4 =       1.513  ;
a5 =     0.08237 ;
b5 =       2.986  ;
c5 =      -1.601  ;
a6 =     0.04641 ;
b6 =       3.964  ;
c6 =       1.738  ;
F_x =   u_VSP*( a1*sin(b1*alpha+c1) + ...
                a2*sin(b2*alpha+c2) + ...
                a3*sin(b3*alpha+c3) + ...
                a4*sin(b4*alpha+c4) + ...
                a5*sin(b5*alpha+c5) + ...
                a6*sin(b6*alpha+c6) );
% Calculating the force in y-direction
a1 =      0.7936 ;
b1 =       1.001  ;
c1 =     0.01605;
a2 =      0.2112 ;
b2 =       1.997  ;
c2 =     0.03229;
a3 =     0.07608;
b3 =       2.991  ;
c3 =       2.986  ;
a4 =     0.04817;
b4 =       3.999  ;
c4 =     -0.8668 ;
a5 =     0.01757;
b5 =       4.904  ;
c5 =      -2.622 ;
a6 =    -0.02089;
b6 =       5.068  ;
c6 =      0.2548 ;
F_y =   u_VSP*( a1*sin(b1*alpha+c1) + ...
                a2*sin(b2*alpha+c2) + ...
                a3*sin(b3*alpha+c3) + ...
                a4*sin(b4*alpha+c4) + ...
                a5*sin(b5*alpha+c5) + ...
                a6*sin(b6*alpha+c6));

== matlab function CSE1_HIL_full16_caseC_new_param/Simulator CSE1/B Command to force mapping/VSP1 ==
  data: alpha input; F_x output; u_VSP input; F_y output
function [ F_x , F_y ] = fcn(alpha,u_VSP)
%#codegen
% Calculating the force in x-direction
a1 =       1.107  ;
b1 =       1.001  ;
c1 =       1.564  ;
a2 =      0.3471 ;
b2 =      0.1397 ;
c2 =      -1.599  ;
a3 =      0.1558 ;
b3 =       1.993  ;
c3 =       1.886  ;
a4 =      0.1599 ;
b4 =       0.218  ;
c4 =       1.513  ;
a5 =     0.08237 ;
b5 =       2.986  ;
c5 =      -1.601  ;
a6 =     0.04641 ;
b6 =       3.964  ;
c6 =       1.738  ;
F_x =   u_VSP*( a1*sin(b1*alpha+c1) + ...
                a2*sin(b2*alpha+c2) + ...
                a3*sin(b3*alpha+c3) + ...
                a4*sin(b4*alpha+c4) + ...
                a5*sin(b5*alpha+c5) + ...
                a6*sin(b6*alpha+c6) );
% Calculating the force in y-direction
a1 =      0.7936 ;
b1 =       1.001  ;
c1 =     0.01605;
a2 =      0.2112 ;
b2 =       1.997  ;
c2 =     0.03229;
a3 =     0.07608;
b3 =       2.991  ;
c3 =       2.986  ;
a4 =     0.04817;
b4 =       3.999  ;
c4 =     -0.8668 ;
a5 =     0.01757;
b5 =       4.904  ;
c5 =      -2.622 ;
a6 =    -0.02089;
b6 =       5.068  ;
c6 =      0.2548 ;
F_y =   u_VSP*( a1*sin(b1*alpha+c1) + ...
                a2*sin(b2*alpha+c2) + ...
                a3*sin(b3*alpha+c3) + ...
                a4*sin(b4*alpha+c4) + ...
                a5*sin(b5*alpha+c5) + ...
                a6*sin(b6*alpha+c6));

== matlab function CSE1_HIL_full16_caseC_new_param/Controller/CtrlCustom_SLX/Observer/Inverse ==
  data: u input; y output
function y = fcn(u)


y = inv(u);

== matlab function CSE1_HIL_full16_caseC_new_param/Controller/CtrlCustom_SLX/Observer/Transpose ==
  data: u input; y output
function y = fcn(u)


y = u.';

== matlab function CSE1_HIL_full16_caseC_new_param/Controller/CtrlCustom_SLX/Control law/Damping and coriolis ==
  data: D output; nu_hat input; C output
function [D,C] = damp_cori_calculator(nu_hat)
%% MATRICES
m = 14.11;   
I_z = 1.7600;
x_g = 0.0375;

%% Added mass
X_ud = -2.0;
Y_vd = -10.0;
N_vd = -0.0;
Y_rd = -0.0;
N_rd = -1.0;
	
%% Damping coefficients
X_u		= -0.6555;
X_uu 	= 0.3545;
X_uuu 	= -3.787;

X_v		= 0;
X_vv	= -2.443;
X_vvv	= 0;

Y_v		= -1.33;
Y_vv	= -2.776;
Y_vvv	= -64.91;

Y_r		= -7.250;
Y_rr	= -3.450;
Y_rrr	= 0;

Y_rv	= -0.805;
Y_vr	= -0.845;

N_v		= 0;
N_vv	= -0.2088;
N_vvv	= 0;

N_r		= -1.900;
N_rr	= -0.750;
N_rrr	= 0;
						
N_rv	= 0.130;
N_vr	= 0.080;

%% Correolis matrix
c_13 = -(m-Y_vd)*nu_hat(2)-(m*x_g-Y_rd)*nu_hat(3);
c_23 = (m-X_ud)*nu_hat(1);

C    = [0       0       c_13;
        0       0       c_23;
        -c_13   -c_23   0   ];
    
%% Assembly of the damping matrix
d_11 = -X_u - X_uu*abs(nu_hat(1)) - X_uuu*nu_hat(1)^2;
d_22 = -Y_v - Y_vv*abs(nu_hat(2)) - Y_vvv*nu_hat(2)^2 - Y_rv*abs(nu_hat(3));
d_33 = -N_r - N_rr*abs(nu_hat(3)) - N_rrr*nu_hat(3)^2 - N_vr*abs(nu_hat(2));

d_23 = -Y_r - Y_rr*abs(nu_hat(3)) - Y_rrr*nu_hat(3)^2 - Y_vr*abs(nu_hat(2));
d_32 = -N_v - N_vv*abs(nu_hat(2)) - N_vvv*nu_hat(2)^2 - N_rv*abs(nu_hat(3));

D    = [d_11    0       0;
        0       d_22    d_23;
        0       d_32    d_33];

== matlab function CSE1_HIL_full16_caseC_new_param/Simulator CSE1/Measurement simulation ==
  data: eta_real input; eta_measured output
function eta_measured = fcn(eta_real)

eta_measured = eta_real;

% atan2(Y,X)
eta_measured(3,1) = atan2(eta_real(2,1),eta_real(1,1));

end

== matlab function CSE1_HIL_full16_caseC_new_param/Round counter/Round counter ==
  data: eta_measured input; eta_adjusted output; eta_measured_prev input; j_prev input; eta_measured_new output; j_new output
function [eta_adjusted, eta_measured_new, j_new] = fcn(eta_measured, eta_measured_prev, j_prev)

if (eta_measured(3,1) - eta_measured_prev(3,1)) < -pi
    j = j_prev + 1;
elseif (eta_measured(3,1) - eta_measured_prev(3,1)) > pi
    j = j_prev - 1;
else
    j = j_prev;
end

eta_adjusted = eta_measured;
eta_adjusted(3,1) = eta_measured(3,1) + 2*pi*j;

eta_measured_new = eta_measured;
j_new = j;

end
